simulink model "DigitalChannel"  (R2023b)
settings: Solver=VariableStepAuto  StartTime=0.0  StopTime=100  RelTol=1e-3
libraries: dspfdesign x1, commsink2 x1, dspsrcs4 x1, dspsigops x1, commrandsrc3 x1

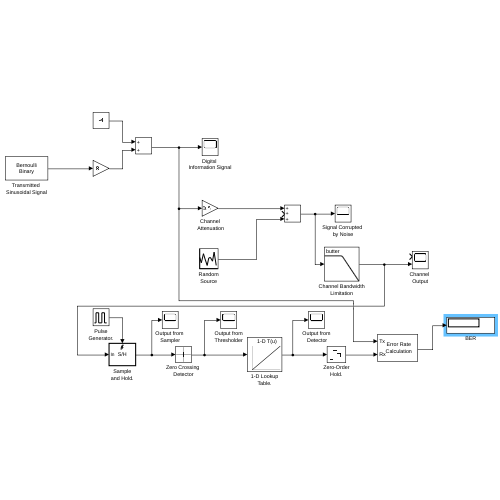
[thumbnail: Simulink's stored preview of the top-level diagram]
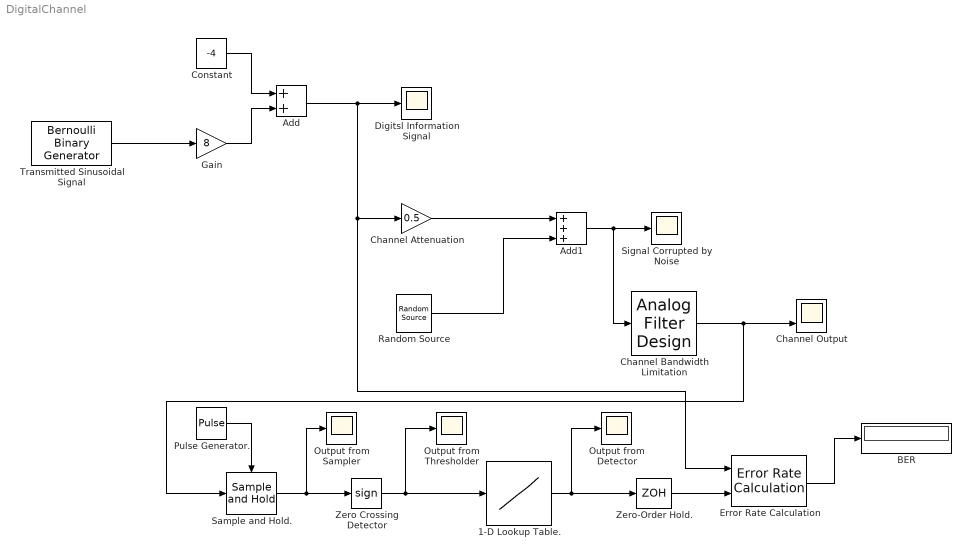
== system DigitalChannel ==
  1-D Lookup Table. : Lookup_n-D  NumberOfTableDimensions=1  BreakpointsForDimension1=[-1,1]  Table=[-4,4]  InternalRulePriority=Speed  RndMeth=Simplest
  Add : Sum
  Add1 : Sum  Inputs=+++
  BER : Display
  Channel Attenuation : Gain  Gain=0.5
  Channel Output : Scope  NumInputPorts=2
  Channel Bandwidth Limitation : dspfdesign/Analog Filter Design  method=Butterworth  filttype=Lowpass  N=10  Wlo=100  Whi=80  Rp=2  Rs=40
  Constant : Constant  Value=-4
  Digitsl Information Signal : Scope
  Error Rate Calculation : commsink2/Error Rate Calculation  N=1  st_delay=0  cp_mode=Entire frame  subframe=[]  PMode=Port  WsName=ErrorVec  RsMode2=off  stop=off  numErr=100  maxBits=1e6
  Gain : Gain  Gain=8
  Output from Detector : Scope
  Output from Thresholder : Scope
  Output from Sampler : Scope
  Pulse Generator. : DiscretePulseGenerator  PulseType=Time based  Period=0.1  PulseWidth=50
  Random Source : dspsrcs4/Random Source  SrcType=Gaussian  NormMethod=Ziggurat  CltLength=12  MinVal=0  MaxVal=1  MeanVal=0  VarVal=1  RepMode=Not repeatable  rawSeed=1  IsInherit=off  SampMode=Discrete  SampTime=0.01  SampFrame=1  DataType=Double  OutComplex=Real  OutputFrames=off
  Sample and Hold. : dspsigops/Sample and Hold  trig=Rising edge  initCond=0  latchinput=off
  Signal Corrupted by Noise : Scope
  Transmitted Sinusoidal Signal : commrandsrc3/Bernoulli Binary Generator  ProbabilityOfZero=0.5  SeedSource=Parameter  Seed=61  SampleTime=0.1  SamplesPerFrame=1  OutputDataType=double  SimulateUsing=Interpreted execution
  Zero Crossing Detector : Signum
  Zero-Order Hold. : ZeroOrderHold  SampleTime=0.1
  wires:
  Transmitted Sinusoidal Signal/1 -> Gain/1
  Gain/1 -> Add/2
  Constant/1 -> Add/1
  Add/1 -> Error Rate Calculation/1, Channel Attenuation/1, Digitsl Information Signal/1
  Channel Attenuation/1 -> Add1/1
  Random Source/1 -> Add1/3
  Add1/1 -> Channel Bandwidth Limitation/1, Signal Corrupted by Noise/1
  Channel Bandwidth Limitation/1 -> Sample and Hold./1, Channel Output/2
  Pulse Generator./1 -> Sample and Hold./Trigger
  Sample and Hold./1 -> Output from Sampler/1, Zero Crossing Detector/1
  Zero Crossing Detector/1 -> Output from Thresholder/1, 1-D Lookup Table./1
  1-D Lookup Table./1 -> Output from Detector/1, Zero-Order Hold./1
  Zero-Order Hold./1 -> Error Rate Calculation/2
  Error Rate Calculation/1 -> BER/1
